simulink model "RETRO_NFB_NON_LIN"  (R2021a)
settings: Solver=VariableStepAuto  StartTime=0.0  StopTime=60  RelTol=1e-3
model workspace (MATLAB code in the model file):
  | Kab=12;
  | Kca=16;
  | Fb=2;
  | Kbc=4;
  | Kcb=25;
  | Kia=8;
  | Fa=6;
  | In=0.3;
  | Kcd=2;
  | Kdc=8;
  | Fd=3;
  | x_star=[0.4000; 0.2360; 0.5000; 0.2500];
settings Model: Creator=priya  LastModifiedBy=Priyan_PC
settings SolverCC: AlgebraicLoopSolver=TrustRegion
settings DebuggingCC: SFMachineParentedDataDiag=warning

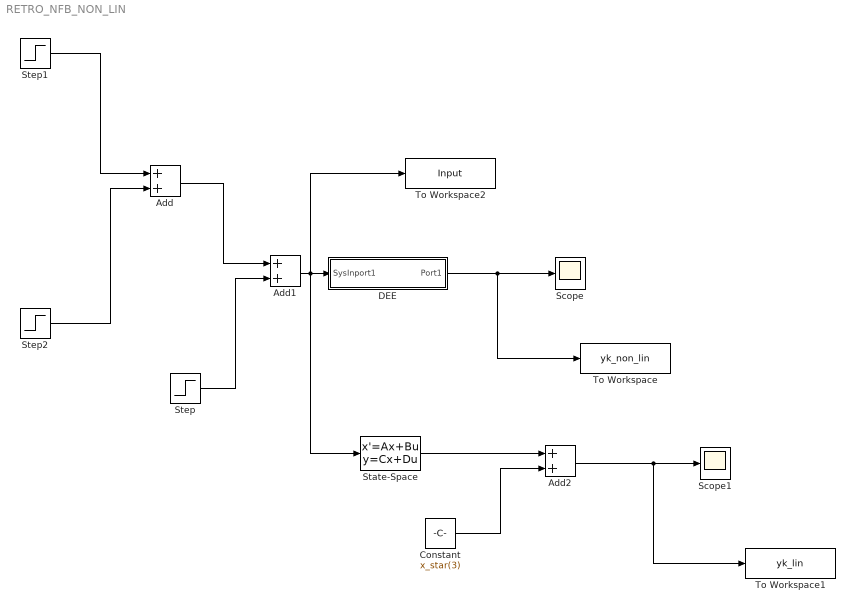
== system RETRO_NFB_NON_LIN ==
  Add : Sum
  Add1 : Sum
  Add2 : Sum
  Constant : Constant  Value=x_star(3)
  DEE : Subsystem  mask(Differential Equation Editor (DEE)){}
      settings: OpenFcn=diffeqed
      mask Display: disp('Differential Equation\n Editor')
  Scope : Scope
  Scope1 : Scope
  State-Space : StateSpace  A=[-6 0 0 0;0 0 4 0;8 -12.5 -12.8 -1;0 0 6 -4]  B=[8;0;0;0]  C=[0 0 1 0]  D=0  InitialCondition=0
  Step : Step  Time=40  After=0.15  SampleTime=0
  Step1 : Step  Time=10  Before=0.3  After=0.5  SampleTime=0
  Step2 : Step  Time=25  After=0.2  SampleTime=0
  To Workspace : ToWorkspace  VariableName=yk_non_lin  SampleTime=-1
  To Workspace1 : ToWorkspace  VariableName=yk_lin  SampleTime=-1
  To Workspace2 : ToWorkspace  VariableName=Input  SampleTime=-1
  wires:
  Step1/1 -> Add/1
  Step/1 -> Add1/2
  Step2/1 -> Add/2
  Add1/1 -> To Workspace2/1, State-Space/1, DEE/1(SysInport1)
  DEE/1(Port1) -> To Workspace/1, Scope/1
  Add/1 -> Add1/1
  State-Space/1 -> Add2/1
  Constant/1 -> Add2/2
  Add2/1 -> To Workspace1/1, Scope1/1

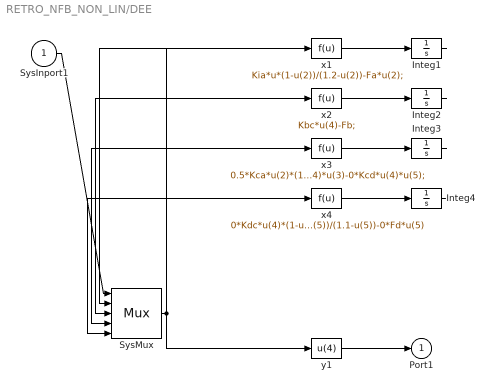
== system RETRO_NFB_NON_LIN/DEE ==
  SysInport1 : Inport
  Integ1 : Integrator  InitialCondition=x_star(1)
  Integ2 : Integrator  InitialCondition=x_star(2)
  Integ3 : Integrator  InitialCondition=x_star(3)
  Integ4 : Integrator  InitialCondition=x_star(4)
  SysMux : Mux  Inputs=5
  x1 : Fcn  Expr=Kia*u*(1-u(2))/(1.2-u(2))-Fa*u(2);
  x2 : Fcn  Expr=Kbc*u(4)-Fb;
  x3 : Fcn  Expr=0.5*Kca*u(2)*(1-u(4))/(1.2-u(4))-0.2*Kcb*u(4)*u(3)-0*Kcd*u(4)*u(5);
  x4 : Fcn  Expr=0*Kdc*u(4)*(1-u(5))/(1.1-u(5))-0*Fd*u(5)
  y1 : Fcn  Expr=u(4)
  Port1 : Outport
  wires:
  SysInport1/1 -> SysMux/1
  SysMux/1 -> x1/1, x2/1, x3/1, x4/1, y1/1
  x1/1 -> Integ1/1
  Integ1/1 -> SysMux/2
  x2/1 -> Integ2/1
  Integ2/1 -> SysMux/3
  x3/1 -> Integ3/1
  Integ3/1 -> SysMux/4
  x4/1 -> Integ4/1
  Integ4/1 -> SysMux/5
  y1/1 -> Port1/1
